simulink model "Lab1PartB1"  (R2023b)
settings: Solver=VariableStepAuto  StartTime=0.0  StopTime=10  RelTol=1e-3
settings Model: Creator=tanvi  LastModifiedBy=tanvi

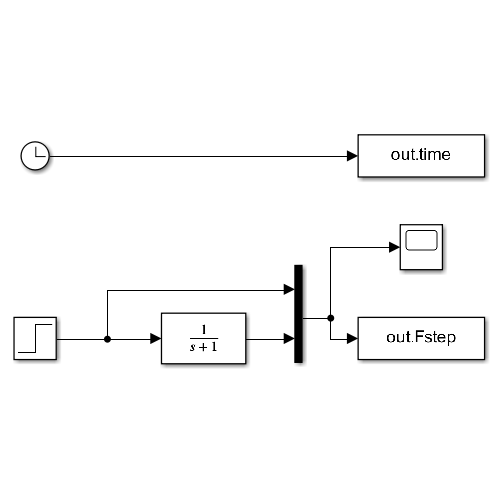
[thumbnail: Simulink's stored preview of the top-level diagram]
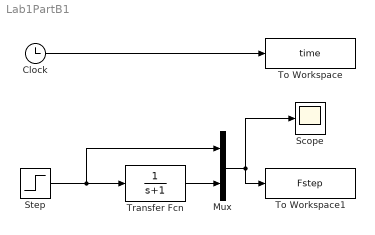
== system Lab1PartB1 ==
  Clock : Clock
  Mux : Mux  Inputs=2
  Scope : Scope
  Step : Step  SampleTime=0
  To Workspace : ToWorkspace  VariableName=time  SaveFormat=Timeseries  SampleTime=-1
  To Workspace1 : ToWorkspace  VariableName=Fstep  SaveFormat=Timeseries  SampleTime=-1
  Transfer Fcn : TransferFcn  Denominator=[1 1]
  wires:
  Step/1 -> Mux/1, Transfer Fcn/1
  Mux/1 -> To Workspace1/1, Scope/1
  Transfer Fcn/1 -> Mux/2
  Clock/1 -> To Workspace/1
